simulink model "model"  (R2015b)
settings: Solver=VariableStepAuto  StartTime=0.0  StopTime=inf  FixedStep=0.0001  RelTol=1e-3
undefined symbols (not defined in the file): B, Jm, Kt, L, R
libraries: fl_lib x5, nesl_utility x3, elec_lib x1, powerlib_meascontrol x1
settings Model: Creator=root  LastModifiedBy=root

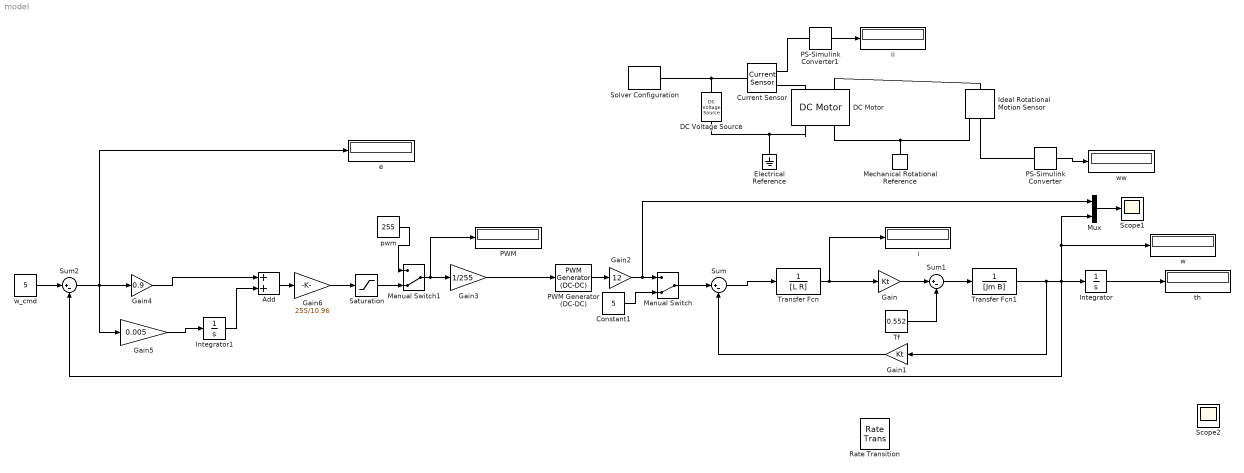
== system model ==
  Add : Sum
  Constant1 : Constant  Value=5
  Current Sensor : fl_lib/Electrical/Electrical Sensors/Current Sensor
  DC Motor : elec_lib/Actuators & Drivers/Rotational Actuators/DC Motor  parameterization=1  Ra=0.457 Ohm  La=0 H  emf_or_torque=1  Kv=1.092 V/(rad/s)  Ki=6.876e-4 N*m/A  T_stall=2.4e-4 N*m  w_max=1.91e+4 rpm  w_rated=1.5e+4 rpm  P_rated=0.08 W  V_rated=1.5 V  J=0.034 kg*m^2  lam_param=1  lam=0.0168 N*m/(rad/s)  i_noload=0 A  V_i_noload=1.5 V  speed0=0 rad/s  alpha=0.00393 1/K  Tmeas=25 C  thermal_mass=100 J/K  initial_temperature=25 C
  DC Voltage Source : fl_lib/Electrical/Electrical Sources/DC Voltage Source  v0=8 V
  Electrical Reference : fl_lib/Electrical/Electrical Elements/Electrical Reference
  Gain : Gain  Gain=Kt
  Gain1 : Gain  Gain=Kt
  Gain2 : Gain  Gain=12
  Gain3 : Gain  Gain=1/255
  Gain4 : Gain  Gain=0.9
  Gain5 : Gain  Gain=0.005
  Gain6 : Gain  Gain=255/10.96
  Ideal Rotational Motion Sensor : fl_lib/Mechanical/Mechanical Sensors/Ideal Rotational Motion Sensor  offset=0 rad
  Integrator : Integrator
  Integrator1 : Integrator
  Manual Switch : ManualSwitch  CurrentSetting=0
  Manual Switch1 : ManualSwitch  CurrentSetting=0
  Mechanical Rotational Reference : fl_lib/Mechanical/Rotational Elements/Mechanical Rotational Reference
  Mux : Mux  Inputs=2
  PS-Simulink Converter : nesl_utility/PS-Simulink Converter  PhysicalDomain=network_engine_domain  SubClassName=ps_output  LeftPortType=input  RightPortType=output  PseudoPeriodic=off  Frequencies=[]  Unit=1  AffineConversion=off
  PS-Simulink Converter1 : nesl_utility/PS-Simulink Converter  PhysicalDomain=network_engine_domain  SubClassName=ps_output  LeftPortType=input  RightPortType=output  PseudoPeriodic=off  Frequencies=[]  Unit=1  AffineConversion=off
  PWM : Display
  PWM Generator (DC-DC) : powerlib_meascontrol/Pulse & Signal Generators/PWM Generator (DC-DC)  Fsw=7812.5  Ts=0
  Rate Transition : RateTransition
  Saturation : Saturate  UpperLimit=255  LowerLimit=-255
  Scope1 : Scope
  Scope2 : Scope
  Solver Configuration : nesl_utility/Solver Configuration  PhysicalDomain=network_engine_domain  SubClassName=solver  LeftPortType=input  RightPortType=generic  Accelerate=off  Tones=[]  Harmonics=[]  SimulateNoise=off  Profile=off  UseLocalSampling=off  EnableSwitchedLinearOptims=on  FrequencyDomain=off  UseCCode=off  RelTol=0.001  AbsTol=1e-06  MinStep=1e-09  ToWorkspace=off  RevertToSquareIcSolve=off  NumHomotopyIterations=100  PhasorMode=off  PhasorModeNumHarmonics=1  DoDC=off  ResidualTolerance=1e-09  UseLocalSolver=off  LocalSolverChoice=NE_BACKWARD_EULER_ADVANCER  LocalSolverSampleTime=0.001  DoFixedCost=off  MaxNonlinIter=3  MaxModeIter=2  LinearAlgebra=Sparse  DelaysMemoryBudget=1024  AutomaticFiltering=on  FilteringTimeConstant=0.001
  Sum : Sum  Inputs=|+-
  Sum1 : Sum  Inputs=|+-
  Sum2 : Sum  Inputs=|+-
  Tf : Constant  Value=0.552
  Transfer Fcn : TransferFcn  Denominator=[L R]
  Transfer Fcn1 : TransferFcn  Denominator=[Jm B]
  e : Display
  i : Display
  ii : Display
  pwm : Constant  Value=255
  th : Display
  w : Display
  w_cmd : Constant  Value=5
  ww : Display
  wires:
  Sum/1 -> Transfer Fcn/1
  Gain1/1 -> Sum/2
  Transfer Fcn/1 -> Gain/1, i/1
  Tf/1 -> Sum1/2
  Sum1/1 -> Transfer Fcn1/1
  Gain/1 -> Sum1/1
  PS-Simulink Converter/1 -> ww/1
  PS-Simulink Converter1/1 -> ii/1
  PWM Generator (DC-DC)/1 -> Gain2/1
  Constant1/1 -> Manual Switch/2
  Gain2/1 -> Mux/1, Manual Switch/1
  Gain3/1 -> PWM Generator (DC-DC)/1
  Manual Switch/1 -> Sum/1
  Mux/1 -> Scope1/1
  Integrator/1 -> th/1
  Manual Switch1/1 -> PWM/1, Gain3/1
  pwm/1 -> Manual Switch1/1
  Gain4/1 -> Add/1
  Transfer Fcn1/1 -> Sum2/2, Mux/2, w/1, Integrator/1, Gain1/1
  Sum2/1 -> e/1, Gain5/1, Gain4/1
  w_cmd/1 -> Sum2/1
  Gain5/1 -> Integrator1/1
  Integrator1/1 -> Add/2
  Add/1 -> Gain6/1
  Saturation/1 -> Manual Switch1/2
  Gain6/1 -> Saturation/1
  connections:
  DC Voltage Source/RConn1 -- DC Motor/RConn1 -- Electrical Reference/LConn1
  DC Voltage Source/LConn1 -- Solver Configuration/RConn1 -- Current Sensor/LConn1
  DC Motor/RConn2 -- Ideal Rotational Motion Sensor/RConn1 -- Mechanical Rotational Reference/LConn1
  DC Motor/LConn2 -- Ideal Rotational Motion Sensor/LConn1
  PS-Simulink Converter/LConn1 -- Ideal Rotational Motion Sensor/RConn2
  Current Sensor/RConn2 -- DC Motor/LConn1
  Current Sensor/RConn1 -- PS-Simulink Converter1/LConn1
